simulink model "ens_IdentificacaoH1H2_Random_v2"  (R2016a)
settings: Solver=ode45  StartTime=0.0  StopTime=7800  RelTol=1e-3
StartFcn:
  | clear all
libraries: realtime_pacer_lib x1
settings Model: Creator=johnh  LastModifiedBy=tiago
settings DataIOCC: SaveFormat=StructureWithTime
settings OptimizationCC: BlockReduction=off  DefaultParameterBehavior=Inlined  BufferReuse=off
settings HardwareCC: ProdWordSize=32  ProdHWDeviceType=Specified
settings ConfigComp: CovModelRefEnable=Off

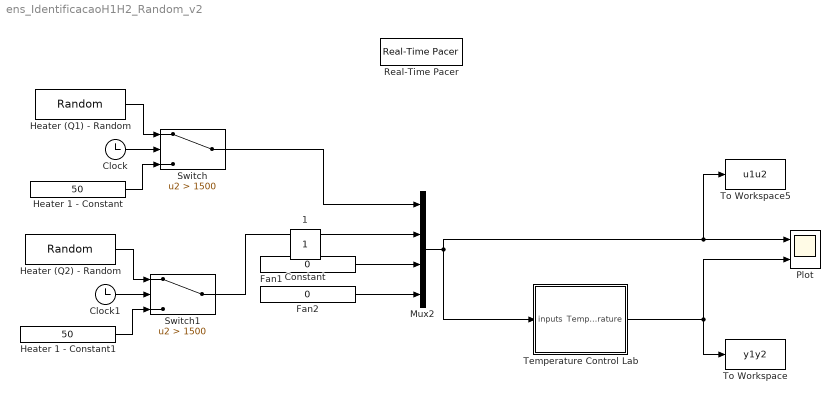
== system ens_IdentificacaoH1H2_Random_v2 ==
  Clock : Clock
  Clock1 : Clock
  Fan1 : Constant  Value=0
  Fan2 : Constant  Value=0
  Heater (Q1) - Random : RandomNumber  Mean=50  Variance=200  Seed=4  SampleTime=105
  Heater (Q2) - Random : RandomNumber  Mean=50  Variance=200  Seed=5  SampleTime=105
  Heater 1 - Constant : Constant  Value=50
  Heater 1 - Constant1 : Constant  Value=50
  Mux2 : Mux
  Plot : Scope  NumInputPorts=2
  Real-Time Pacer : realtime_pacer_lib/Real-Time Pacer  simTimePerRealTime=1
  Switch : Switch  Criteria=u2 > Threshold  Threshold=1500
  Switch1 : Switch  Criteria=u2 > Threshold  Threshold=1500
  Temperature Control Lab : Subsystem
      mask Display: image('tclab.png');
  To Workspace : ToWorkspace  VariableName=y1y2  SaveFormat=Timeseries  SampleTime=-1
  To Workspace5 : ToWorkspace  VariableName=u1u2  SaveFormat=Timeseries  SampleTime=-1
  1 : Constant  IOType=siggen
  Constant : Constant  IOType=siggen
  wires:
  Temperature Control Lab/1(Temperature) -> Plot/2, To Workspace/1
  Mux2/1 -> To Workspace5/1, Plot/1, Temperature Control Lab/1(inputs)
  Fan1/1 -> Mux2/3
  Fan2/1 -> Mux2/4
  Clock/1 -> Switch/2
  Switch/1 -> Mux2/1
  Heater (Q1) - Random/1 -> Switch/1
  Heater 1 - Constant/1 -> Switch/3
  Clock1/1 -> Switch1/2
  Switch1/1 -> Mux2/2
  Heater (Q2) - Random/1 -> Switch1/1
  Heater 1 - Constant1/1 -> Switch1/3

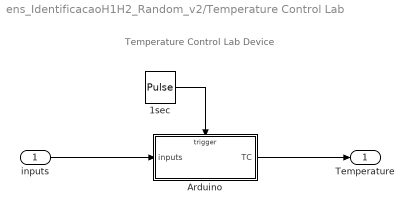
== system ens_IdentificacaoH1H2_Random_v2/Temperature Control Lab ==
  note: Temperature Control Lab Device
  inputs : Inport
  1sec : DiscretePulseGenerator  PulseType=Time based  Period=0.5  PulseWidth=50
  Arduino : Subsystem  TreatAsAtomicUnit=on
  Temperature : Outport
  wires:
  1sec/1 -> Arduino/Trigger
  Arduino/1(TC) -> Temperature/1
  inputs/1 -> Arduino/1(inputs)

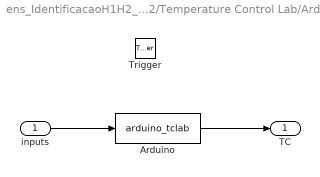
== system ens_IdentificacaoH1H2_Random_v2/Temperature Control Lab/Arduino ==
  inputs : Inport  LatchByDelayingOutsideSignal=on
  Trigger : TriggerPort  VariantControl=Variant
  Arduino : MATLABFcn  MATLABFcn=arduino_tclab
  TC : Outport  InitialOutput=[23 23]
  wires:
  inputs/1 -> Arduino/1
  Arduino/1 -> TC/1
